simulink model "ApproachModel_PitchHold"  (R2017a)
settings: Solver=VariableStepAuto  StartTime=0.0  StopTime=70  RelTol=1e-3
libraries: cstblocks x2, simulink x1
settings Model: Creator=user  LastModifiedBy=user

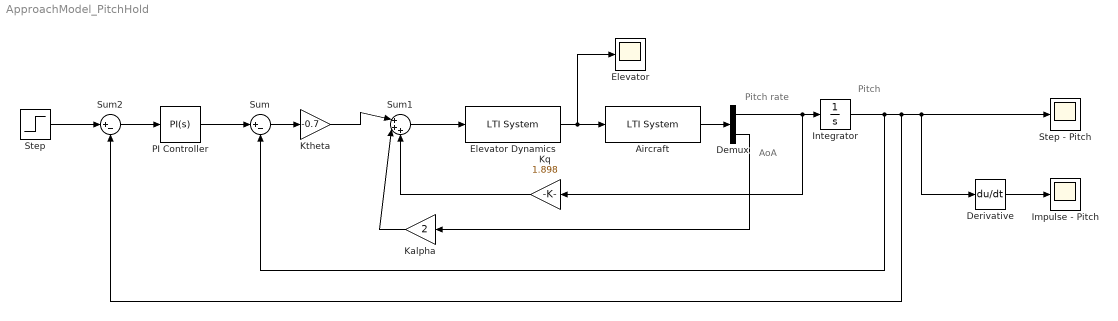
== system ApproachModel_PitchHold ==
  note: AoA
  note: Pitch
  note: Pitch rate
  Aircraft : cstblocks/LTI System  sys=Sys1  IC=[]
  Demux : Demux  Outputs=2
  Derivative : Derivative
  Elevator : Scope
  "Elevator Dynamics " : cstblocks/LTI System  sys=tf(10,[1 10])  IC=[]
  Impulse - Pitch : Scope
  Integrator : Integrator
  Kalpha : Gain  Gain=2
  Kq : Gain  Gain=1.898
  Ktheta : Gain  Gain=-0.7
  PI Controller : simulink/Continuous/PID Controller  Controller=PI  TimeDomain=Continuous-time  SampleTime=-1  IntegratorMethod=Forward Euler  FilterMethod=Forward Euler  Form=Parallel  UseFilter=on  ControllerParametersSource=internal  P=0.5  I=0.7  D=0  N=100  InitialConditionSource=internal  InitialConditionForIntegrator=0  InitialConditionForFilter=0  ExternalReset=none  LimitOutput=off  UpperSaturationLimit=inf  LowerSaturationLimit=-inf  LinearizeAsGain=on  AntiWindupMode=none  Kb=1  TrackingMode=off  Kt=1  PParamMin=[]  PParamMax=[]  IParamMin=[]  IParamMax=[]  DParamMin=[]  DParamMax=[]  NParamMin=[]  NParamMax=[]  KbParamMin=[]  KbParamMax=[]  KtParamMin=[]  KtParamMax=[]  POutMin=[]  POutMax=[]  IOutMin=[]  IOutMax=[]  DOutMin=[]  DOutMax=[]  NOutMin=[]  NOutMax=[]  KbOutMin=[]  KbOutMax=[]  KtOutMin=[]  KtOutMax=[]  IntegratorOutMin=[]  IntegratorOutMax=[]  FilterOutMin=[]  FilterOutMax=[]  SumOutMin=[]  SumOutMax=[]  SumI1OutMin=[]  SumI1OutMax=[]  SumI2OutMin=[]  SumI2OutMax=[]  SumI3OutMin=[]  SumI3OutMax=[]  SumDOutMin=[]  SumDOutMax=[]  SaturationOutMin=[]  SaturationOutMax=[]  IntegratorContinuousStateAttributes=''  IntegratorStateMustResolveToSignalObject=off  IntegratorRTWStateStorageClass=Auto  FilterContinuousStateAttributes=''  FilterStateMustResolveToSignalObject=off  FilterRTWStateStorageClass=Auto  DifferentiatorICPrevScaledInput=0  DifferentiatorOutMin=[]  DifferentiatorOutMax=[]  InitialConditionSetting=State (most efficient)
  Step : Step  Time=0  SampleTime=0
  Step - Pitch : Scope
  Sum : Sum  Inputs=|+-
  Sum1 : Sum  Inputs=|+++
  Sum2 : Sum  Inputs=|+-
  wires:
  Integrator/1 -> Sum2/2, Derivative/1, Step - Pitch/1, Sum/2
  "Elevator Dynamics "/1 -> Elevator/1, Aircraft/1
  Demux/1 -> Kq/1, Integrator/1
  Aircraft/1 -> Demux/1
  Demux/2 -> Kalpha/1
  Sum1/1 -> "Elevator Dynamics "/1
  Kalpha/1 -> Sum1/2
  Sum/1 -> Ktheta/1
  Derivative/1 -> Impulse - Pitch/1
  Kq/1 -> Sum1/3
  Ktheta/1 -> Sum1/1
  Sum2/1 -> PI Controller/1
  Step/1 -> Sum2/1
  PI Controller/1 -> Sum/1
